simulink model "lab5"  (R2019b)
settings: Solver=VariableStepAuto  StartTime=0.0  StopTime=10.0  RelTol=1e-3
settings Model: NumberOfSteps=10  Creator=1  LastModifiedBy=1

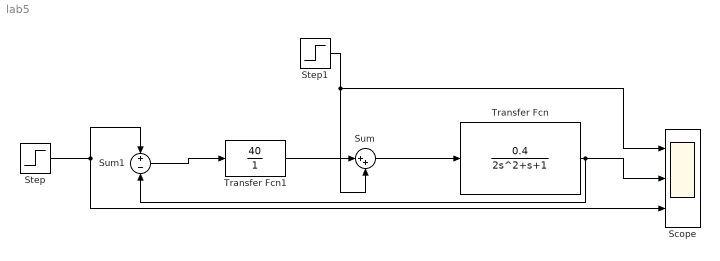
== system lab5 ==
  Scope : Scope  NumInputPorts=3
  Step : Step  SampleTime=0
  Step1 : Step  SampleTime=0
  Sum : Sum  Inputs=|++
  Sum1 : Sum  Inputs=+-
  Transfer Fcn : TransferFcn  Numerator=[0.4]  Denominator=[2 1 1]
  Transfer Fcn1 : TransferFcn  Numerator=[40]  Denominator=[1]
  wires:
  Sum/1 -> Transfer Fcn/1
  Step1/1 -> Scope/1, Sum/2
  Transfer Fcn1/1 -> Sum/1
  Step/1 -> Scope/3, Sum1/1
  Transfer Fcn/1 -> Sum1/2, Scope/2
  Sum1/1 -> Transfer Fcn1/1
